simulink model "LMPC_all"  (R2019a)
settings: Solver=FixedStepAuto  StartTime=0.0  StopTime=3  RelTol=1e-3
undefined symbols (not defined in the file): Cf, Cr, Iz, lf, lr, m
libraries: mpclib x4
settings Model: Creator=Johan PC  LastModifiedBy=Johan PC
settings DataIOCC: ReturnWorkspaceOutputs=off
settings OptimizationCC: DefaultParameterBehavior=Inlined  EnhancedBackFolding=on  PassReuseOutputArgsAs=Individual arguments  OptimizeBlockOrder=speed  DifferentSizesBufferReuse=on
settings DebuggingCC: ParameterTunabilityLossMsg=error  ArithmeticOperatorsInVariantConditions=warning
settings SFSimCC: MATLABDynamicMemAlloc=off
settings RTWCC: SystemTargetFile=ert.tlc  TemplateMakefile=ert_default_tmf  GenerateReport=on  IncludeHyperlinkInReport=on  LaunchReport=on  GenerateTraceInfo=on  GenerateTraceReport=on  GenerateTraceReportSl=on  GenerateTraceReportSf=on  GenerateTraceReportEml=on
settings CodeAppCC: ForceParamTrailComments=on  IgnoreCustomStorageClasses=off  OperatorAnnotations=on  SimulinkDataObjDesc=on  SFDataObjDesc=on  InsertBlockDesc=on
settings ERTTargetCC: TargetLangStandard=C99 (ISO)  GenerateSampleERTMain=on  InlinedParameterPlacement=NonHierarchical  RTWCAPISignals=on  ERTCustomFileTemplate=example_file_process.tlc

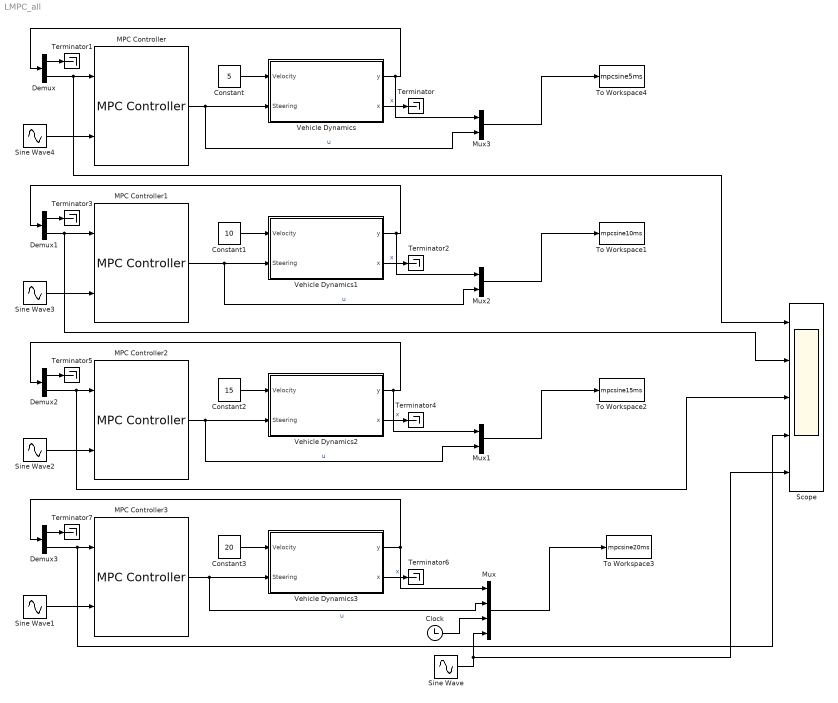
== system LMPC_all ==
  Clock : Clock
  Constant : Constant  Value=5
  Constant1 : Constant  Value=10
  Constant2 : Constant  Value=15
  Constant3 : Constant  Value=20
  Demux{,1..3} (4 alike) : Demux  Outputs=2
  MPC Controller{,1..3} (4 alike) : mpclib/MPC Controller  SCDEnableBlockLinearizationSpecification=on  mpcobj=mpc1a  is_multiple=0  enable_value=0  return_u0=off  updateMPCinCallerWorkspace=on  md_inport=off  mv_inport=off  uref_inport=off  return_cost=off  return_mvseq=off  return_qpstatus=off  return_xseq=off  return_state=off  return_ovseq=off  state_inport=off  umin_inport=off  umax_inport=off  ymin_inport=off  ymax_inport=off  cc_inport=off  ywt_inport=off  uwt_inport=off  duwt_inport=off  rhoeps_inport=off  pm_inport=off  MaximumP=10  HorizonChoice=FixedHorizon  n_ts=0.01  n_p=10  n_mv=1  n_md=0  n_ud=0  n_mo=1  n_uo=0  BlockDataType=double  SampleTimeInherited=off  switch_inport=off
  Mux : Mux
  Mux1 : Mux  Inputs=2
  Mux2 : Mux  Inputs=2
  Mux3 : Mux  Inputs=2
  Scope : Scope  NumInputPorts=5
  Sine Wave{,1..4} (5 alike) : Sin  Amplitude=2  Frequency=2  SampleTime=0
  Terminator{,1..7} (8 alike) : Terminator
  To Workspace1 : ToWorkspace  VariableName=mpcsine10ms  SampleTime=-1
      settings: Save2DSignal=2-D array (concatenate along first dimension)
  To Workspace2 : ToWorkspace  VariableName=mpcsine15ms  SampleTime=-1
      settings: Save2DSignal=2-D array (concatenate along first dimension)
  To Workspace3 : ToWorkspace  VariableName=mpcsine20ms  SampleTime=-1
      settings: Save2DSignal=2-D array (concatenate along first dimension)
  To Workspace4 : ToWorkspace  VariableName=mpcsine5ms  SampleTime=-1
      settings: Save2DSignal=2-D array (concatenate along first dimension)
  Vehicle Dynamics : Subsystem
  Vehicle Dynamics1 : Subsystem
  Vehicle Dynamics2 : Subsystem
  Vehicle Dynamics3 : Subsystem
  wires:
  Sine Wave4/1 -> MPC Controller/2
  Constant/1 -> Vehicle Dynamics/1(Velocity)
  Vehicle Dynamics/2(x) -> Terminator/1  "x"
  Demux/2 -> Scope/1, MPC Controller/1
  Demux/1 -> Terminator1/1
  Demux1/1 -> Terminator3/1
  Vehicle Dynamics1/2(x) -> Terminator2/1  "x"
  Sine Wave3/1 -> MPC Controller1/2
  Constant1/1 -> Vehicle Dynamics1/1(Velocity)
  Demux1/2 -> Scope/2, MPC Controller1/1
  Demux2/1 -> Terminator5/1
  Vehicle Dynamics2/2(x) -> Terminator4/1  "x"
  Sine Wave2/1 -> MPC Controller2/2
  Constant2/1 -> Vehicle Dynamics2/1(Velocity)
  Demux2/2 -> Scope/3, MPC Controller2/1
  Vehicle Dynamics3/1("y ") -> Demux3/1, Mux/1
  Demux3/1 -> Terminator7/1
  Vehicle Dynamics3/2(x) -> Terminator6/1  "x"
  Sine Wave1/1 -> MPC Controller3/2
  Constant3/1 -> Vehicle Dynamics3/1(Velocity)
  MPC Controller3/1 -> Mux/2, Vehicle Dynamics3/2(Steering)  "u"
  Demux3/2 -> Scope/4, MPC Controller3/1
  Mux/1 -> To Workspace3/1
  Mux1/1 -> To Workspace2/1
  Vehicle Dynamics2/1("y ") -> Mux1/1, Demux2/1
  MPC Controller2/1 -> Mux1/2, Vehicle Dynamics2/2(Steering)  "u"
  Mux2/1 -> To Workspace1/1
  Vehicle Dynamics1/1("y ") -> Mux2/1, Demux1/1
  MPC Controller1/1 -> Mux2/2, Vehicle Dynamics1/2(Steering)  "u"
  Mux3/1 -> To Workspace4/1
  Vehicle Dynamics/1("y ") -> Mux3/1, Demux/1
  MPC Controller/1 -> Mux3/2, Vehicle Dynamics/2(Steering)  "u"
  Clock/1 -> Mux/3
  Sine Wave/1 -> Scope/5, Mux/4

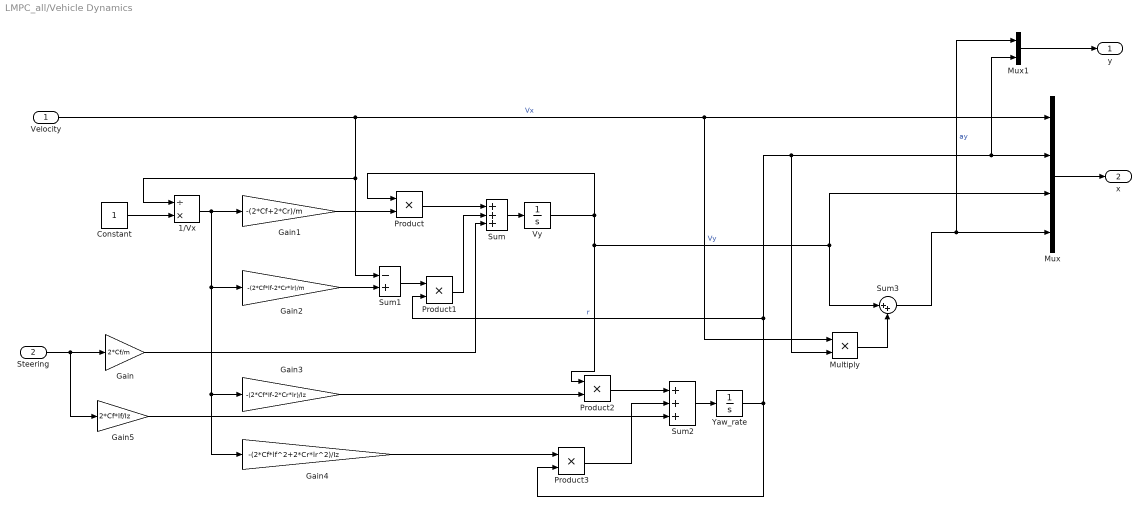
== system LMPC_all/Vehicle Dynamics ==
  Velocity : Inport
  Steering : Inport  Port=2
  1/Vx : Product  Inputs=/*
  Constant : Constant
  Gain : Gain  Gain=2*Cf/m
  Gain1 : Gain  Gain=-(2*Cf+2*Cr)/m
  Gain2 : Gain  Gain=-(2*Cf*lf-2*Cr*lr)/m
  Gain3 : Gain  Gain=-(2*Cf*lf-2*Cr*lr)/Iz
  Gain4 : Gain  Gain=-(2*Cf*lf^2+2*Cr*lr^2)/Iz
  Gain5 : Gain  Gain=2*Cf*lf/Iz
  Multiply : Product
  Mux : Mux
  Mux1 : Mux  Inputs=2
  Product{,1..3} (4 alike) : Product
  Sum : Sum  Inputs=+++
  Sum1 : Sum  Inputs=-+
  Sum2 : Sum  Inputs=+++
  Sum3 : Sum  Inputs=|++
  Vy : Integrator
  "Yaw_rate " : Integrator
  "y " : Outport
  x : Outport  Port=2
  wires:
  Sum2/1 -> "Yaw_rate "/1
  Gain2/1 -> Sum1/2
  Gain4/1 -> Product3/1
  Constant/1 -> 1/Vx/2
  Gain3/1 -> Product2/2
  1/Vx/1 -> Gain4/1, Gain3/1, Gain2/1, Gain1/1
  Product2/1 -> Sum2/1
  Product3/1 -> Sum2/2
  Gain5/1 -> Sum2/3
  Sum1/1 -> Product1/1
  "Yaw_rate "/1 -> Multiply/2, Mux1/2, Mux/2, Product1/2, Product3/2  "r"
  Gain/1 -> Sum/3
  Steering/1 -> Gain/1, Gain5/1
  Gain1/1 -> Product/2
  Product/1 -> Sum/1
  Vy/1 -> Product2/1, Mux/3, Sum3/1, Product/1  "Vy"
  Sum/1 -> Vy/1
  Velocity/1 -> Mux/1, Multiply/1, 1/Vx/1, Sum1/1  "Vx"
  Product1/1 -> Sum/2
  Multiply/1 -> Sum3/2
  Sum3/1 -> Mux1/1, Mux/4  "ay"
  Mux/1 -> x/1
  Mux1/1 -> "y "/1

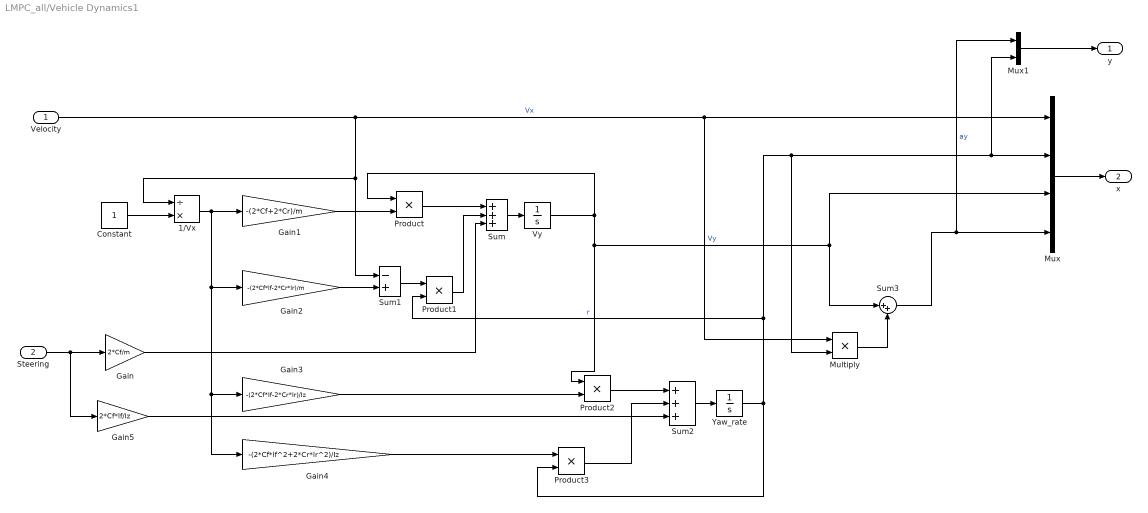
== system LMPC_all/Vehicle Dynamics1 ==
  Velocity : Inport
  Steering : Inport  Port=2
  1/Vx : Product  Inputs=/*
  Constant : Constant
  Gain : Gain  Gain=2*Cf/m
  Gain1 : Gain  Gain=-(2*Cf+2*Cr)/m
  Gain2 : Gain  Gain=-(2*Cf*lf-2*Cr*lr)/m
  Gain3 : Gain  Gain=-(2*Cf*lf-2*Cr*lr)/Iz
  Gain4 : Gain  Gain=-(2*Cf*lf^2+2*Cr*lr^2)/Iz
  Gain5 : Gain  Gain=2*Cf*lf/Iz
  Multiply : Product
  Mux : Mux
  Mux1 : Mux  Inputs=2
  Product{,1..3} (4 alike) : Product
  Sum : Sum  Inputs=+++
  Sum1 : Sum  Inputs=-+
  Sum2 : Sum  Inputs=+++
  Sum3 : Sum  Inputs=|++
  Vy : Integrator
  "Yaw_rate " : Integrator
  "y " : Outport
  x : Outport  Port=2
  wires:
  Sum2/1 -> "Yaw_rate "/1
  Gain2/1 -> Sum1/2
  Gain4/1 -> Product3/1
  Constant/1 -> 1/Vx/2
  Gain3/1 -> Product2/2
  1/Vx/1 -> Gain4/1, Gain3/1, Gain2/1, Gain1/1
  Product2/1 -> Sum2/1
  Product3/1 -> Sum2/2
  Gain5/1 -> Sum2/3
  Sum1/1 -> Product1/1
  "Yaw_rate "/1 -> Multiply/2, Mux1/2, Mux/2, Product1/2, Product3/2  "r"
  Gain/1 -> Sum/3
  Steering/1 -> Gain/1, Gain5/1
  Gain1/1 -> Product/2
  Product/1 -> Sum/1
  Vy/1 -> Product2/1, Mux/3, Sum3/1, Product/1  "Vy"
  Sum/1 -> Vy/1
  Velocity/1 -> Mux/1, Multiply/1, 1/Vx/1, Sum1/1  "Vx"
  Product1/1 -> Sum/2
  Multiply/1 -> Sum3/2
  Sum3/1 -> Mux1/1, Mux/4  "ay"
  Mux/1 -> x/1
  Mux1/1 -> "y "/1

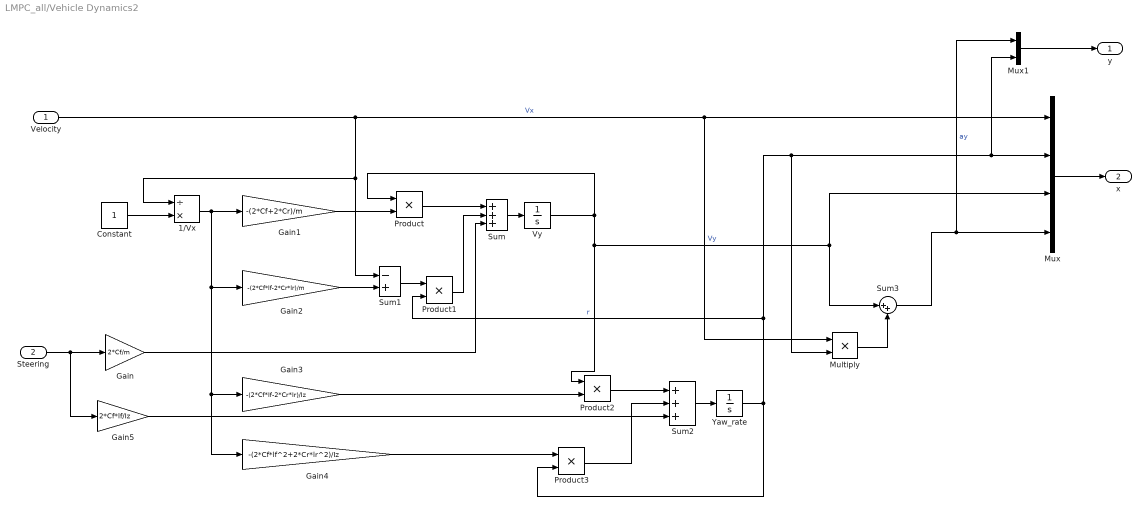
== system LMPC_all/Vehicle Dynamics2 ==
  Velocity : Inport
  Steering : Inport  Port=2
  1/Vx : Product  Inputs=/*
  Constant : Constant
  Gain : Gain  Gain=2*Cf/m
  Gain1 : Gain  Gain=-(2*Cf+2*Cr)/m
  Gain2 : Gain  Gain=-(2*Cf*lf-2*Cr*lr)/m
  Gain3 : Gain  Gain=-(2*Cf*lf-2*Cr*lr)/Iz
  Gain4 : Gain  Gain=-(2*Cf*lf^2+2*Cr*lr^2)/Iz
  Gain5 : Gain  Gain=2*Cf*lf/Iz
  Multiply : Product
  Mux : Mux
  Mux1 : Mux  Inputs=2
  Product{,1..3} (4 alike) : Product
  Sum : Sum  Inputs=+++
  Sum1 : Sum  Inputs=-+
  Sum2 : Sum  Inputs=+++
  Sum3 : Sum  Inputs=|++
  Vy : Integrator
  "Yaw_rate " : Integrator
  "y " : Outport
  x : Outport  Port=2
  wires:
  Sum2/1 -> "Yaw_rate "/1
  Gain2/1 -> Sum1/2
  Gain4/1 -> Product3/1
  Constant/1 -> 1/Vx/2
  Gain3/1 -> Product2/2
  1/Vx/1 -> Gain4/1, Gain3/1, Gain2/1, Gain1/1
  Product2/1 -> Sum2/1
  Product3/1 -> Sum2/2
  Gain5/1 -> Sum2/3
  Sum1/1 -> Product1/1
  "Yaw_rate "/1 -> Multiply/2, Mux1/2, Mux/2, Product1/2, Product3/2  "r"
  Gain/1 -> Sum/3
  Steering/1 -> Gain/1, Gain5/1
  Gain1/1 -> Product/2
  Product/1 -> Sum/1
  Vy/1 -> Product2/1, Mux/3, Sum3/1, Product/1  "Vy"
  Sum/1 -> Vy/1
  Velocity/1 -> Mux/1, Multiply/1, 1/Vx/1, Sum1/1  "Vx"
  Product1/1 -> Sum/2
  Multiply/1 -> Sum3/2
  Sum3/1 -> Mux1/1, Mux/4  "ay"
  Mux/1 -> x/1
  Mux1/1 -> "y "/1

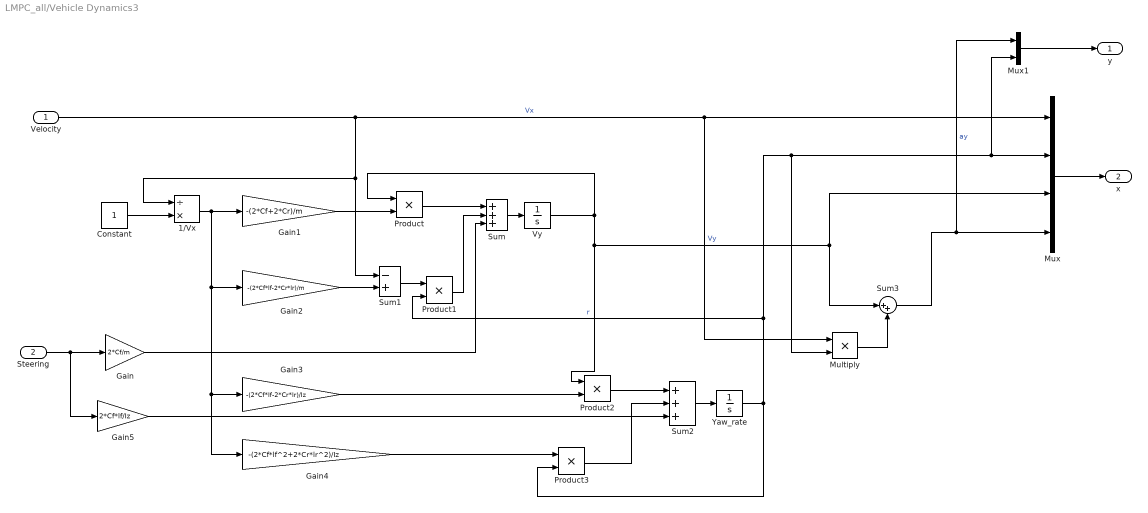
== system LMPC_all/Vehicle Dynamics3 ==
  Velocity : Inport
  Steering : Inport  Port=2
  1/Vx : Product  Inputs=/*
  Constant : Constant
  Gain : Gain  Gain=2*Cf/m
  Gain1 : Gain  Gain=-(2*Cf+2*Cr)/m
  Gain2 : Gain  Gain=-(2*Cf*lf-2*Cr*lr)/m
  Gain3 : Gain  Gain=-(2*Cf*lf-2*Cr*lr)/Iz
  Gain4 : Gain  Gain=-(2*Cf*lf^2+2*Cr*lr^2)/Iz
  Gain5 : Gain  Gain=2*Cf*lf/Iz
  Multiply : Product
  Mux : Mux
  Mux1 : Mux  Inputs=2
  Product{,1..3} (4 alike) : Product
  Sum : Sum  Inputs=+++
  Sum1 : Sum  Inputs=-+
  Sum2 : Sum  Inputs=+++
  Sum3 : Sum  Inputs=|++
  Vy : Integrator
  "Yaw_rate " : Integrator
  "y " : Outport
  x : Outport  Port=2
  wires:
  Sum2/1 -> "Yaw_rate "/1
  Gain2/1 -> Sum1/2
  Gain4/1 -> Product3/1
  Constant/1 -> 1/Vx/2
  Gain3/1 -> Product2/2
  1/Vx/1 -> Gain4/1, Gain3/1, Gain2/1, Gain1/1
  Product2/1 -> Sum2/1
  Product3/1 -> Sum2/2
  Gain5/1 -> Sum2/3
  Sum1/1 -> Product1/1
  "Yaw_rate "/1 -> Multiply/2, Mux1/2, Mux/2, Product1/2, Product3/2  "r"
  Gain/1 -> Sum/3
  Steering/1 -> Gain/1, Gain5/1
  Gain1/1 -> Product/2
  Product/1 -> Sum/1
  Vy/1 -> Product2/1, Mux/3, Sum3/1, Product/1  "Vy"
  Sum/1 -> Vy/1
  Velocity/1 -> Mux/1, Multiply/1, 1/Vx/1, Sum1/1  "Vx"
  Product1/1 -> Sum/2
  Multiply/1 -> Sum3/2
  Sum3/1 -> Mux1/1, Mux/4  "ay"
  Mux/1 -> x/1
  Mux1/1 -> "y "/1
